simulink model "zynqRadioHWSWQPSKAD9361AD9364SL"  (R2016a)
settings: Solver=FixedStepDiscrete  SolverMode=SingleTasking  StartTime=0.0  StopTime=inf  RelTol=1e-3
PreLoadFcn:
  | % Ensure SDR libraries are added to path
  | tempradiodev_ = sdrdev('ZC706 and FMCOMMS2/3/4');
  | tempradiodev_.setupSession();
  | clear tempradiodev_; % clean up
  | 
  | sdrzQPSKTxFPGA_params = zynqRadioQPSKTxFPGAAD9361AD9364SL_init;
  | sdrzQPSKrxFPGA = zynqRadioQPSKRxFPGAAD9361AD9364SL_init;
  | 
  | % Need preamble & data from CST's QPSK Tx HDL example
  | qpsktxhdl=commqpsktxhdl_init();
  | 
  | % ARM Tx message
  | txtstr = '*Zynq HW/SW Codesign*';
InitFcn:
  | sdrzQPSKTxFPGA_params = zynqRadioQPSKTxFPGAAD9361AD9364SL_init;
  | sdrzQPSKrxFPGA = zynqRadioQPSKRxFPGAAD9361AD9364SL_init;
  | 
  | % Need preamble & data from CST's QPSK Tx HDL example
  | qpsktxhdl=commqpsktxhdl_init();
  | 
  | if (numel(txtstr) > 24)
  |   error('txtstr message must be less than 24 characters');
  | end;
undefined symbols (not defined in the file or in its folder): msglen
libraries: hdlsllib x9, dspsigops x7, commsequence2 x2, commdigbbndpm3 x2, dspmlti4 x2, commrandsrc2 x1, commutil2 x1, simulink x1, dspmathops x1
(part 1 of 2)
CloseFcn:
  | clear qpsktxhdl sdrzQPSKrxFPGA sdrzQPSKTxFPGA_params txtstr;
settings Model: DataTypeOverride=Off  Creator=The MathWorks, Inc.  LastModifiedBy=The MathWorks, Inc.
settings DataIOCC: SaveFormat=Array  SaveOutput=off  SaveTime=off
settings OptimizationCC: BlockReduction=off  ConditionallyExecuteInputs=off  DefaultParameterBehavior=Inlined
settings DebuggingCC: AlgebraicLoopMsg=error  SolverPrmCheckMsg=warning  SingleTaskRateTransMsg=error  ParameterPrecisionLossMsg=none  StrictBusMsg=ErrorOnBusTreatedAsVector
settings HardwareCC: ProdBitPerPointer=32  ProdLargestAtomicFloat=None  ProdIntDivRoundTo=Undefined  ProdEndianess=Unspecified  ProdWordSize=32  ProdHWDeviceType=ASIC/FPGA->ASIC/FPGA  ProdEqTarget=off
settings ModelReferenceCC: PropagateSignalLabelsOutOfModel=off

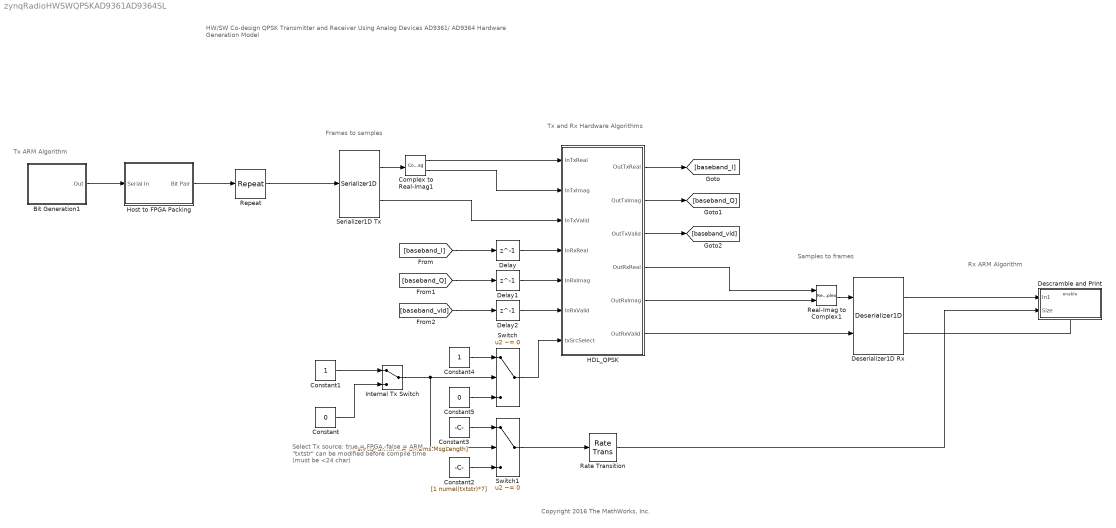
== system zynqRadioHWSWQPSKAD9361AD9364SL ==
  note: Select Tx source:
      | true = FPGA, false = ARM
      |
      | "txtstr" can be modified before
      | compile time (must be <24 char)
  note: Tx and Rx Hardware Algorithms
  note: HW/SW Co-design QPSK Transmitter and Receiver Using Analog Devices AD9361/ AD9364
      | Hardware Generation Model
  note: Rx ARM Algorithm
  note: Samples to frames
  note: Frames to samples
  note: Tx ARM Algorithm
  note: Copyright 2016 The MathWorks, Inc.
  Bit Generation1 : Subsystem
      mask Display: disp('Bits Generation')
  Complex to Real-Imag1 : ComplexToRealImag
  Constant : Constant  Value=0  OutDataTypeStr=boolean  SampleTime=-1
  Constant1 : Constant  OutDataTypeStr=boolean  SampleTime=-1
  Constant2 : Constant  Value=[1 numel(txtstr)*7]  SampleTime=-1
  Constant3 : Constant  Value=[1 sdrzQPSKTxFPGA_params.MsgLength]  SampleTime=-1
  Constant4 : Constant  OutDataTypeStr=boolean  SampleTime=-1
  Constant5 : Constant  Value=0  OutDataTypeStr=boolean  SampleTime=-1
  Delay : Delay  DelayLength=1
  Delay1 : Delay  DelayLength=1
  Delay2 : Delay  DelayLength=1
  Descramble and Print : Subsystem  TreatAsAtomicUnit=on
  Deserializer1D Rx : hdlsllib/HDL Operations/Deserializer1D  Ratio=sdrzQPSKrxFPGA.FrameSize  IdleCycles=0  InitialCondition=0  startIn=off  validIn=on  validOut=on  inputDataDimensions=-1  inputSampleTime=-1  inputSignalType=auto
  HDL_QPSK : Subsystem  TreatAsAtomicUnit=on
  Host to FPGA Packing : Subsystem
  Internal Tx Switch : ManualSwitch
  Rate Transition : RateTransition
  Real-Imag to Complex1 : RealImagToComplex
  Repeat : dspsigops/Repeat  N=4  InputProcessing=Columns as channels (frame based)  RateOptions=Allow multirate processing  ic=0  mode=Unused parameter value
  Serializer1D Tx : hdlsllib/HDL Operations/Serializer1D  Ratio=200  IdleCycles=0  validIn=off  startOut=off  validOut=on  inputDataDimensions=-1  inputSampleTime=-1  inputSignalType=auto
  Switch : Switch  Criteria=u2 ~= 0
  Switch1 : Switch  Criteria=u2 ~= 0
  wires:
  Deserializer1D Rx/1 -> Descramble and Print/1(In1)
  Real-Imag to Complex1/1 -> Deserializer1D Rx/1
  Deserializer1D Rx/2 -> Descramble and Print/Enable
  HDL_QPSK/4(OutRxReal) -> Real-Imag to Complex1/1
  HDL_QPSK/5(OutRxImag) -> Real-Imag to Complex1/2
  HDL_QPSK/6(OutRxValid) -> Deserializer1D Rx/2
  HDL_QPSK/1(OutTxReal) -> [baseband_I]
  HDL_QPSK/2(OutTxImag) -> [baseband_Q]
  HDL_QPSK/3(OutTxValid) -> [baseband_vld]
  [baseband_I] -> Delay/1
  [baseband_Q] -> Delay1/1
  [baseband_vld] -> Delay2/1
  Delay/1 -> HDL_QPSK/4(InRxReal)
  Delay1/1 -> HDL_QPSK/5(InRxImag)
  Delay2/1 -> HDL_QPSK/6(InRxValid)
  Host to FPGA Packing/1(Bit Pair) -> Repeat/1
  Bit Generation1/1(Out) -> Host to FPGA Packing/1(Serial In)
  Repeat/1 -> Serializer1D Tx/1
  Serializer1D Tx/1 -> Complex to Real-Imag1/1
  Complex to Real-Imag1/1 -> HDL_QPSK/1(InTxReal)
  Complex to Real-Imag1/2 -> HDL_QPSK/2(InTxImag)
  Serializer1D Tx/2 -> HDL_QPSK/3(InTxValid)
  Constant/1 -> Internal Tx Switch/2
  Constant1/1 -> Internal Tx Switch/1
  Switch1/1 -> Rate Transition/1
  Switch/1 -> HDL_QPSK/7(txSrcSelect)
  Internal Tx Switch/1 -> Switch1/2, Switch/2
  Constant4/1 -> Switch/1
  Constant5/1 -> Switch/3
  Constant2/1 -> Switch1/3
  Constant3/1 -> Switch1/1
  Rate Transition/1 -> Descramble and Print/2(Size)

== system zynqRadioHWSWQPSKAD9361AD9364SL/Bit Generation1 ==
  note: Each data frame contains 26 bits header (For Sync Purpose) and 174 bits data bits which
      | contain the txtStr message.Scrambler is there to improve data transition density and
      |  frequency offset estimation.
  Barker Code SS : Subsystem
      mask Display: disp('Unipolar\nBarker Code')
  Frame Conversion : FrameConversion  InheritSamplingMode=off  OutFrame=Sample-based
  Matrix Concatenate : Concatenate  Mode=Multidimensional array
  Message Source : Subsystem
      mask Display: disp('Message\nSource')
  Repeat : dspsigops/Repeat  N=2  InputProcessing=Columns as channels (frame based)  RateOptions=Enforce single-rate processing  ic=0  mode=Unused parameter value
  Scrambler : commsequence2/Scrambler  M=2  poly=[1 1 1 0 1]  iniStaSource=Dialog Parameter  ini_sta=[0 0 0 0]  resetViaPort=off
  Out : Outport
  wires:
  Message Source/1(Out) -> Scrambler/1
  Scrambler/1 -> Matrix Concatenate/2
  Repeat/1 -> Matrix Concatenate/1
  Barker Code SS/1(Out) -> Repeat/1
  Matrix Concatenate/1 -> Frame Conversion/1
  Frame Conversion/1 -> Out/1

== system zynqRadioHWSWQPSKAD9361AD9364SL/Descramble and Print ==
  In1 : Inport
  Size : Inport  Port=2
  Enable : EnablePort  PropagateVarSize=During execution
  BitsToDecimal1 : MATLAB Function  TreatAsAtomicUnit=on
  DataFramer : MATLAB Function  TreatAsAtomicUnit=on
  Descrambling : Subsystem
      mask Display: disp('Descrambling')
  wires:
  DataFramer/1(dataOut) -> Descrambling/1(In)
  In1/1 -> DataFramer/1(dataIn)
  Descrambling/1(Out) -> BitsToDecimal1/1(u)
  Size/1 -> Descrambling/2(Size)

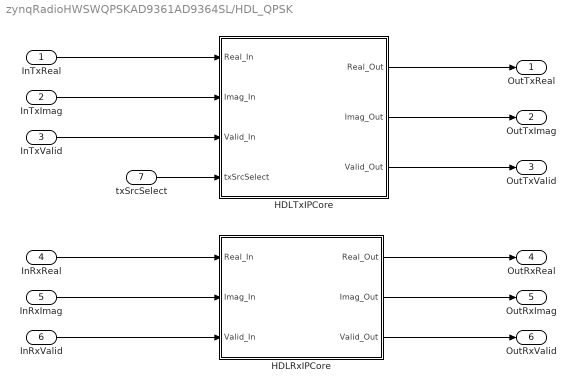
== system zynqRadioHWSWQPSKAD9361AD9364SL/HDL_QPSK ==
  InTxReal : Inport
  InTxImag : Inport  Port=2
  InTxValid : Inport  Port=3
  InRxReal : Inport  Port=4
  InRxImag : Inport  Port=5
  InRxValid : Inport  Port=6
  txSrcSelect : Inport  Port=7
  HDLRxIPCore : Subsystem  TreatAsAtomicUnit=on
  HDLTxIPCore : Subsystem  TreatAsAtomicUnit=on
  OutTxReal : Outport
  OutTxImag : Outport  Port=2
  OutTxValid : Outport  Port=3
  OutRxReal : Outport  Port=4
  OutRxImag : Outport  Port=5
  OutRxValid : Outport  Port=6
  wires:
  HDLTxIPCore/2(Imag_Out) -> OutTxImag/1
  InRxValid/1 -> HDLRxIPCore/3(Valid_In)
  HDLRxIPCore/3(Valid_Out) -> OutRxValid/1
  HDLRxIPCore/2(Imag_Out) -> OutRxImag/1
  HDLRxIPCore/1(Real_Out) -> OutRxReal/1
  HDLTxIPCore/3(Valid_Out) -> OutTxValid/1
  InRxImag/1 -> HDLRxIPCore/2(Imag_In)
  InRxReal/1 -> HDLRxIPCore/1(Real_In)
  HDLTxIPCore/1(Real_Out) -> OutTxReal/1
  InTxReal/1 -> HDLTxIPCore/1(Real_In)
  InTxImag/1 -> HDLTxIPCore/2(Imag_In)
  InTxValid/1 -> HDLTxIPCore/3(Valid_In)
  txSrcSelect/1 -> HDLTxIPCore/4(txSrcSelect)

== system zynqRadioHWSWQPSKAD9361AD9364SL/Host to FPGA Packing ==
  Serial In : Inport
  Data Type Conversion1 : DataTypeConversion  OutDataTypeStr=int16
  Downsample : DownSample  RateOptions=Allow multirate processing
  Downsample1 : DownSample  phase=1  RateOptions=Allow multirate processing
  Real-Imag to Complex : RealImagToComplex
  Bit Pair : Outport
  wires:
  Downsample/1 -> Real-Imag to Complex/1
  Serial In/1 -> Data Type Conversion1/1
  Data Type Conversion1/1 -> Downsample1/1, Downsample/1
  Downsample1/1 -> Real-Imag to Complex/2
  Real-Imag to Complex/1 -> Bit Pair/1

== system zynqRadioHWSWQPSKAD9361AD9364SL/Bit Generation1/Barker Code SS ==
  Constant Barker Code : Constant  Value=|  VectorParams1D=off  OutDataTypeStr=double
      | [+1 +1 +1 +1 +1 -1 -1 +1 +1 -1 +1 -1 +1
      | ].' > 0  % Bipolar to Unipolar Conversion
  Out : Outport
  wires:
  Constant Barker Code/1 -> Out/1

== system zynqRadioHWSWQPSKAD9361AD9364SL/Bit Generation1/Message Source ==
  Bernoulli Binary Generator : commrandsrc2/Bernoulli Binary Generator  P=0.5  seed=61  Ts=sdrzQPSKTxFPGA_params.FrameTime / (sdrzQPSKTxFPGA_params.DataLength - numel(txtstr)*7)  frameBased=on  sampPerFrame=sdrzQPSKTxFPGA_params.DataLength - numel(txtstr)*7  orient=off  outDataType=double
  Integer to Bit Converter : commutil2/Integer to Bit Converter  nbits=7  signedInputValues=Unsigned  bitOrder=MSB first  outDtype=Inherit via internal rule
  Matrix Concatenate : Concatenate  Mode=Multidimensional array
  Scroll text : Constant  Value=double(txtstr)
  Out : Outport
  wires:
  Matrix Concatenate/1 -> Out/1
  Bernoulli Binary Generator/1 -> Matrix Concatenate/2
  Integer to Bit Converter/1 -> Matrix Concatenate/1
  Scroll text/1 -> Integer to Bit Converter/1

== system zynqRadioHWSWQPSKAD9361AD9364SL/Descramble and Print/Descrambling ==
  In : Inport
  Size : Inport  Port=2
  Descrambler : commsequence2/Descrambler  M=2  poly=[1 1 1 0 1]  iniStaSource=Dialog Parameter  ini_sta=[0 0 0 0]  resetViaPort=off
  Selector : Selector  IndexOptions=Index vector (dialog)  Indices=[sdrzQPSKrxFPGA.BarkerLength*log2(sdrzQPSKrxFPGA.M)+1:sdrzQPSKrxFPGA.FrameSize*log2(sdrzQPSKrxFPGA.M)]  OutputSizes=1
  Selector1 : Selector  IndexOptions=Starting and ending indices (port)  Indices=[1:msglen]  OutputSizes=1
  Out : Outport
  wires:
  Selector/1 -> Descrambler/1
  In/1 -> Selector/1
  Selector1/1 -> Out/1
  Descrambler/1 -> Selector1/1
  Size/1 -> Selector1/2

== system zynqRadioHWSWQPSKAD9361AD9364SL/HDL_QPSK/HDLRxIPCore ==
  Real_In : Inport
  Imag_In : Inport  Port=2
  Valid_In : Inport  Port=3
  Complex to Real-Imag1 : ComplexToRealImag
  Enabled Delay : Delay  DelayLength=1  ShowEnablePort=on
      settings: InputPortMap=u0,e6
  HDLRx : Subsystem
  Real-Imag to Complex : RealImagToComplex
  Repeat : dspsigops/Repeat  N=sdrzQPSKrxFPGA.Upsampling/sdrzQPSKrxFPGA.Downsampling  InputProcessing=Inherited (this choice will be removed - see release notes)  RateOptions=Allow multirate processing  ic=0  mode=Unused parameter value
  Upsample : dspsigops/Upsample  N=sdrzQPSKrxFPGA.Upsampling/sdrzQPSKrxFPGA.Downsampling  phase=0  InputProcessing=Inherited (this choice will be removed - see release notes)  RateOptions=Allow multirate processing  ic=0  mode=Unused parameter value
  Real_Out : Outport
  Imag_Out : Outport  Port=2
  Valid_Out : Outport  Port=3
  wires:
  HDLRx/2(dValidOut) -> Upsample/1
  Upsample/1 -> Valid_Out/1
  Repeat/1 -> Complex to Real-Imag1/1
  Complex to Real-Imag1/1 -> Real_Out/1
  Valid_In/1 -> Enabled Delay/2
  Complex to Real-Imag1/2 -> Imag_Out/1
  HDLRx/1(dataOutCh1) -> Repeat/1
  Real-Imag to Complex/1 -> Enabled Delay/1
  Enabled Delay/1 -> HDLRx/1(dataInCh1)
  Real_In/1 -> Real-Imag to Complex/1
  Imag_In/1 -> Real-Imag to Complex/2

== system zynqRadioHWSWQPSKAD9361AD9364SL/HDL_QPSK/HDLTxIPCore ==
  Real_In : Inport
  Imag_In : Inport  Port=2
  Valid_In : Inport  Port=3
  txSrcSelect : Inport  Port=4
  Complex to Real-Imag1 : ComplexToRealImag
  Delay : Delay  DelayLength=1
  Enabled Delay : Delay  DelayLength=1  ShowEnablePort=on
      settings: InputPortMap=u0,e6
  HDLTx : Subsystem
  Real-Imag to Complex : RealImagToComplex
  Real_Out : Outport
  Imag_Out : Outport  Port=2
  Valid_Out : Outport  Port=3
  wires:
  Complex to Real-Imag1/1 -> Real_Out/1
  Complex to Real-Imag1/2 -> Imag_Out/1
  HDLTx/1(dataoutCh1) -> Complex to Real-Imag1/1
  HDLTx/2(validoutCh1) -> Valid_Out/1
  Real-Imag to Complex/1 -> Enabled Delay/1
  Valid_In/1 -> HDLTx/2(validInCh1), Enabled Delay/2
  Real_In/1 -> Real-Imag to Complex/1
  Imag_In/1 -> Real-Imag to Complex/2
  Enabled Delay/1 -> HDLTx/1(dataInCh1)
  txSrcSelect/1 -> Delay/1
  Delay/1 -> HDLTx/3(txSrcSelect)

== system zynqRadioHWSWQPSKAD9361AD9364SL/HDL_QPSK/HDLRxIPCore/HDLRx ==
  dataInCh1 : Inport
  Automatic Gain Control : Subsystem  mask{AGCLoopGain=0.1, AGCUpperLimit=400, AGCRef=1/sqrt(sdrzQPSKrxFPGA.Upsampling)}
      mask prompts: AGCLoopGain "Loop Gain"; AGCUpperLimit "Maximum Gain"; AGCRef "Desired Amplitude"
  Coarse Frequency Compensation : Subsystem
  Data Decoding : Subsystem  TreatAsAtomicUnit=on  mask{Threshold=16}
      mask help:
      | Package synchronization is achieved by correlating (matched filtering) the Barker codes with the streams given by the Timing Recovery subsystem.
      | We deem successful package synchronization if the modulus of the matched filter output exceeds the threshold value defined below.
  FPGA to Host : Subsystem
  Fine Frequency Compensation : Subsystem
  Logical Operator1 : Logic  AllPortsSameDT=off  OutDataTypeStr=boolean
  Raised Cosine Receive Filter : dspmlti4/FIR Decimation  FilterSource=Dialog parameters  h=sdrzQPSKrxFPGA.ReceiverFilterCoefficients  D=sdrzQPSKrxFPGA.Upsampling/sdrzQPSKrxFPGA.Downsampling  filtStruct=Direct form  FilterObject=Hm_firdecim  framing=Allow multirate processing  inputOffset=0  outputBufInitCond=0  roundingMode=Floor  overflowMode=off  firstCoeffDataTypeStr=Inherit: Same word length as input  firstCoeffMin=[]  firstCoeffMax=[]  firstCoeffLastDataTypeStr=Inherit: Same word length as input  outputMode=Binary point scaling  outputWordLength=16  outputFracLength=14  outputDataTypeStr=fixdt(1,16,14)  outputMin=[]  outputMax=[]  outputLastDataTypeStr=fixdt(1,16,14)
  Timing Recovery : Subsystem
  dataOutCh1 : Outport
  dValidOut : Outport  Port=2
  wires:
  Logical Operator1/1 -> dValidOut/1
  Raised Cosine Receive Filter/1 -> Coarse Frequency Compensation/1(In)
  Automatic Gain Control/1(Out) -> Raised Cosine Receive Filter/1
  FPGA to Host/1(Out) -> dataOutCh1/1
  Data Decoding/2(Bit1) -> FPGA to Host/1(bit1)
  Data Decoding/3(Bit2) -> FPGA to Host/2(bit2)
  Data Decoding/1(dValid) -> Logical Operator1/2
  Timing Recovery/1(dValid) -> Data Decoding/Enable, Logical Operator1/1
  Coarse Frequency Compensation/1(Out) -> Fine Frequency Compensation/1(In)
  Fine Frequency Compensation/1(Out) -> Timing Recovery/1(In)
  dataInCh1/1 -> Automatic Gain Control/1(In)
  Timing Recovery/2(DataOut) -> Data Decoding/1(In)

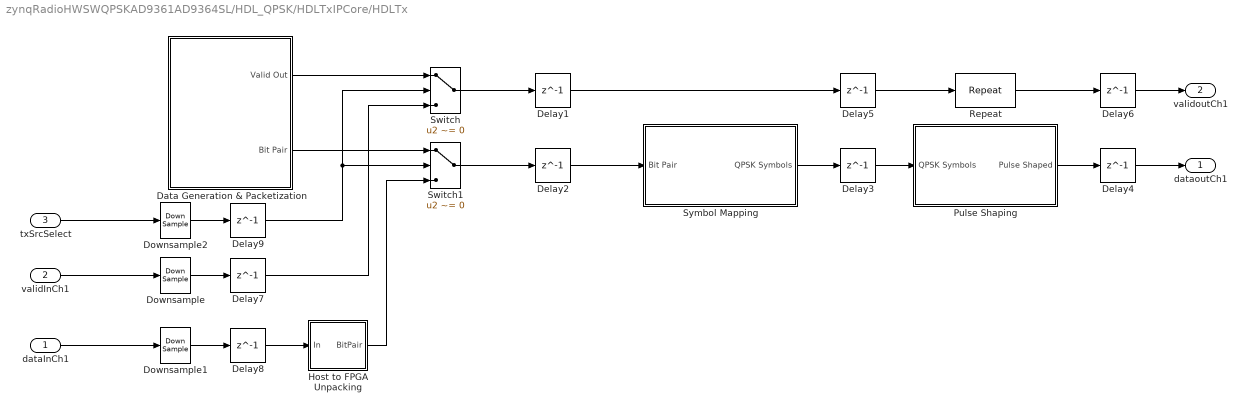
== system zynqRadioHWSWQPSKAD9361AD9364SL/HDL_QPSK/HDLTxIPCore/HDLTx ==
  dataInCh1 : Inport
  validInCh1 : Inport  Port=2
  txSrcSelect : Inport  Port=3
  Data Generation & Packetization : Subsystem
  Delay{1..9} (9 alike) : Delay  DelayLength=1  InitialCondition=0
  Downsample : DownSample  N=sdrzQPSKTxFPGA_params.Upsampling  RateOptions=Allow multirate processing
  Downsample1 : DownSample  N=sdrzQPSKTxFPGA_params.Upsampling  RateOptions=Allow multirate processing
  Downsample2 : DownSample  N=sdrzQPSKTxFPGA_params.Upsampling  RateOptions=Allow multirate processing
  Host to FPGA Unpacking : Subsystem
  Pulse Shaping : Subsystem
  Repeat : dspsigops/Repeat  N=sdrzQPSKTxFPGA_params.Upsampling  InputProcessing=Inherited (this choice will be removed - see release notes)  RateOptions=Allow multirate processing  ic=0  mode=Unused parameter value
  Switch : Switch  Criteria=u2 ~= 0
  Switch1 : Switch  Criteria=u2 ~= 0
  Symbol Mapping : Subsystem
  dataoutCh1 : Outport
  validoutCh1 : Outport  Port=2
  wires:
  Delay3/1 -> Pulse Shaping/1(QPSK Symbols)
  Pulse Shaping/1(Pulse Shaped) -> Delay4/1
  Delay4/1 -> dataoutCh1/1
  Delay2/1 -> Symbol Mapping/1(Bit Pair)
  Symbol Mapping/1(QPSK Symbols) -> Delay3/1
  Delay1/1 -> Delay5/1
  Delay5/1 -> Repeat/1
  Repeat/1 -> Delay6/1
  Delay6/1 -> validoutCh1/1
  Data Generation & Packetization/1(Valid Out) -> Switch/1
  Data Generation & Packetization/2(Bit Pair) -> Switch1/1
  Switch/1 -> Delay1/1
  Switch1/1 -> Delay2/1
  Downsample/1 -> Delay7/1
  Downsample1/1 -> Delay8/1
  validInCh1/1 -> Downsample/1
  dataInCh1/1 -> Downsample1/1
  Delay8/1 -> Host to FPGA Unpacking/1(In)
  Host to FPGA Unpacking/1(BitPair) -> Switch1/3
  Delay7/1 -> Switch/3
  Downsample2/1 -> Delay9/1
  txSrcSelect/1 -> Downsample2/1
  Delay9/1 -> Switch/2, Switch1/2

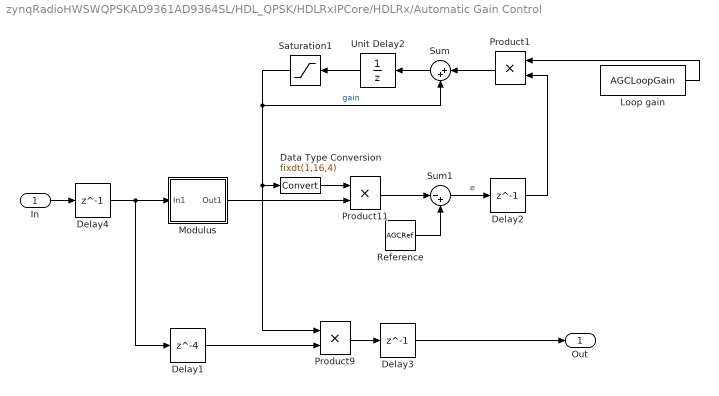
== system zynqRadioHWSWQPSKAD9361AD9364SL/HDL_QPSK/HDLRxIPCore/HDLRx/Automatic Gain Control ==
  In : Inport
  Data Type Conversion : DataTypeConversion  OutDataTypeStr=fixdt(1,16,4)  SaturateOnIntegerOverflow=on
  Delay1 : Delay  DelayLength=4  InitialCondition=0
  Delay2 : Delay  DelayLength=1  InitialCondition=0
  Delay3 : Delay  DelayLength=1  InitialCondition=0
  Delay4 : Delay  DelayLength=1  InitialCondition=0
  Loop gain : Constant  Value=AGCLoopGain  OutDataTypeStr=fixdt(1,16,10)  SampleTime=sdrzQPSKrxFPGA.Ts
  Modulus : Subsystem
  Product1 : Product  OutDataTypeStr=fixdt(1,16,10)  RndMeth=Zero
  Product11 : Product  OutDataTypeStr=fixdt(1,16,10)  RndMeth=Zero
  Product9 : Product  OutDataTypeStr=fixdt(1,16,14)  SaturateOnIntegerOverflow=on  RndMeth=Zero
  Reference : Constant  Value=AGCRef  OutDataTypeStr=fixdt(1,16,10)  SampleTime=sdrzQPSKrxFPGA.Ts
  Saturation1 : Saturate  UpperLimit=AGCUpperLimit  LowerLimit=1e-5
  Sum : Sum  Inputs=|++  OutDataTypeStr=fixdt(1,23,10)  SaturateOnIntegerOverflow=on
  Sum1 : Sum  Inputs=|-+  OutDataTypeStr=Inherit: Same as first input
  Unit Delay2 : UnitDelay  SampleTime=-1
  Out : Outport  PortDimensions=1
  wires:
  Loop gain/1 -> Product1/1
  Saturation1/1 -> Product9/1, Data Type Conversion/1, Sum/2  "gain"
  Product1/1 -> Sum/1
  Modulus/1(Out1) -> Product11/2
  Delay4/1 -> Modulus/1(In1), Delay1/1
  Unit Delay2/1 -> Saturation1/1
  Delay2/1 -> Product1/2
  Delay3/1 -> Out/1
  Delay1/1 -> Product9/2
  Product9/1 -> Delay3/1
  Sum1/1 -> Delay2/1  "e"
  Sum/1 -> Unit Delay2/1
  Reference/1 -> Sum1/2
  Data Type Conversion/1 -> Product11/1
  Product11/1 -> Sum1/1
  In/1 -> Delay4/1

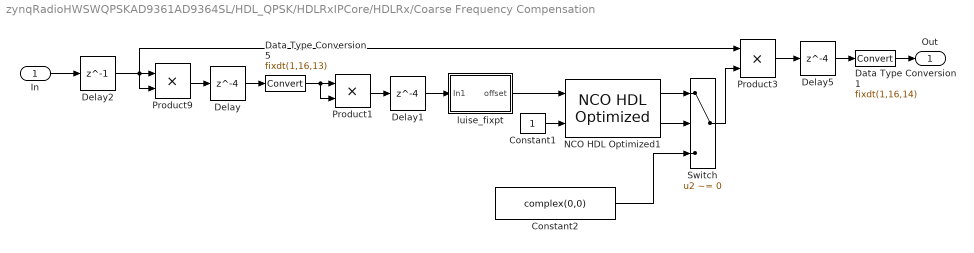
== system zynqRadioHWSWQPSKAD9361AD9364SL/HDL_QPSK/HDLRxIPCore/HDLRx/Coarse Frequency Compensation ==
  In : Inport  PortDimensions=1
  Constant1 : Constant  OutDataTypeStr=boolean  SampleTime=sdrzQPSKrxFPGA.Ts*sdrzQPSKrxFPGA.Upsampling/sdrzQPSKrxFPGA.Downsampling
  Constant2 : Constant  Value=complex(0,0)  OutDataTypeStr=fixdt(1,10,8)  SampleTime=sdrzQPSKrxFPGA.Ts*sdrzQPSKrxFPGA.Upsampling/sdrzQPSKrxFPGA.Downsampling
  Data Type Conversion1 : DataTypeConversion  OutDataTypeStr=fixdt(1,16,14)
  Data Type Conversion5 : DataTypeConversion  OutDataTypeStr=fixdt(1,16,13)  SaturateOnIntegerOverflow=on
  Delay : Delay  DelayLength=4  InitialCondition=0
  Delay1 : Delay  DelayLength=4  InitialCondition=0
  Delay2 : Delay  DelayLength=1  InitialCondition=0
  Delay5 : Delay  DelayLength=4  InitialCondition=0
  NCO HDL Optimized1 : dspsigops/NCO HDL Optimized  PhaseIncrementSource=Input port  PhaseIncrement=100  PhaseOffsetSource=Property  PhaseOffset=0  DitherSource=None  NumDitherBits=1  PhaseQuantization=on  NumQuantizerAccumulatorBits=16  LUTCompress=on  ResetAction=off  ValidInputPort=on  Waveform=Complex exponential  PhasePort=off  AccumulatorWL=17  OutputDataType=Binary point scaling  OutputWL=10  OutputFL=8  SimulateUsing=Code generation
  Product1 : Product  SaturateOnIntegerOverflow=on  RndMeth=Zero
  Product3 : Product  SaturateOnIntegerOverflow=on  RndMeth=Zero
  Product9 : Product  SaturateOnIntegerOverflow=on  RndMeth=Zero
  Switch : Switch  Criteria=u2 ~= 0
  luise_fixpt : Subsystem
  Out : Outport
  wires:
  luise_fixpt/1(offset) -> NCO HDL Optimized1/1
  Delay2/1 -> Product9/1, Product9/2, Product3/1
  Switch/1 -> Product3/2
  Constant2/1 -> Switch/3
  NCO HDL Optimized1/1 -> Switch/1
  NCO HDL Optimized1/2 -> Switch/2
  Constant1/1 -> NCO HDL Optimized1/2
  Delay5/1 -> Data Type Conversion1/1
  Product3/1 -> Delay5/1
  In/1 -> Delay2/1
  Product1/1 -> Delay1/1
  Data Type Conversion5/1 -> Product1/2, Product1/1
  Delay/1 -> Data Type Conversion5/1
  Product9/1 -> Delay/1
  Delay1/1 -> luise_fixpt/1(In1)
  Data Type Conversion1/1 -> Out/1

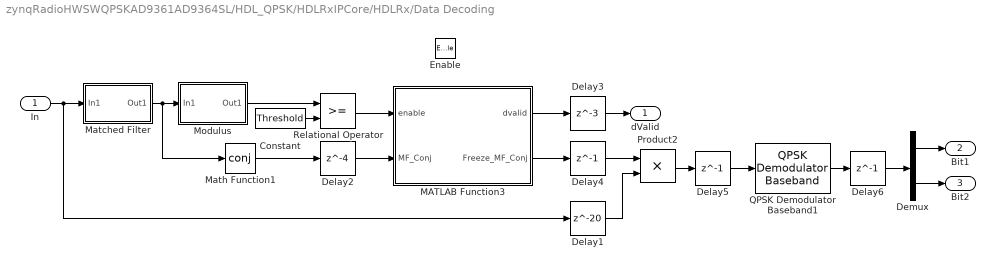
== system zynqRadioHWSWQPSKAD9361AD9364SL/HDL_QPSK/HDLRxIPCore/HDLRx/Data Decoding ==
  In : Inport
  Enable : EnablePort
  Constant : Constant  Value=Threshold  OutDataTypeStr=Inherit: Inherit via back propagation  SampleTime=sdrzQPSKrxFPGA.Ts*sdrzQPSKrxFPGA.Upsampling/sdrzQPSKrxFPGA.Downsampling
  Delay1 : Delay  DelayLength=20  InitialCondition=0
  Delay2 : Delay  DelayLength=4  InitialCondition=0
  Delay3 : Delay  DelayLength=3  InitialCondition=0
  Delay4 : Delay  DelayLength=1  InitialCondition=0
  Delay5 : Delay  DelayLength=1  InitialCondition=0
  Delay6 : Delay  DelayLength=1  InitialCondition=0
  Demux : Demux  Outputs=2
  MATLAB Function3 : MATLAB Function  TreatAsAtomicUnit=on
  Matched Filter : Subsystem
  Math Function1 : Math  Operator=conj  OutputSignalType=complex  SaturateOnIntegerOverflow=on
  Modulus : Subsystem
  Product2 : Product  SaturateOnIntegerOverflow=on  RndMeth=Zero
  QPSK Demodulator Baseband1 : commdigbbndpm3/QPSK Demodulator Baseband  OutType=Bit  DecType=Hard decision  VarSource=Dialog  Variance=1  Dec=Gray  Ph=pi/4  outDtype1=boolean  outDtype2=Inherit via internal rule  derotateFactorWordLen=16  derotateFactorDataTypeStr=Inherit: Same word length as input  derotateFactorLastDataTypeStr=Inherit: Same word length as input
  Relational Operator : RelationalOperator  OutDataTypeStr=boolean  InputSameDT=on
  dValid : Outport  InitialOutput=0
  Bit1 : Outport  Port=2  InitialOutput=0
  Bit2 : Outport  Port=3  InitialOutput=0
  wires:
  Constant/1 -> Relational Operator/2
  Modulus/1(Out1) -> Relational Operator/1
  QPSK Demodulator Baseband1/1 -> Delay6/1
  MATLAB Function3/1(dvalid) -> Delay3/1
  MATLAB Function3/2(Freeze_MF_Conj) -> Delay4/1
  Math Function1/1 -> Delay2/1
  Relational Operator/1 -> MATLAB Function3/1(enable)
  Product2/1 -> Delay5/1
  In/1 -> Matched Filter/1(In1), Delay1/1
  Matched Filter/1(Out1) -> Modulus/1(In1), Math Function1/1
  Delay2/1 -> MATLAB Function3/2(MF_Conj)
  Delay4/1 -> Product2/1
  Delay1/1 -> Product2/2
  Delay5/1 -> QPSK Demodulator Baseband1/1
  Delay6/1 -> Demux/1
  Delay3/1 -> dValid/1
  Demux/1 -> Bit1/1
  Demux/2 -> Bit2/1

== system zynqRadioHWSWQPSKAD9361AD9364SL/HDL_QPSK/HDLRxIPCore/HDLRx/FPGA to Host ==
  bit1 : Inport
  bit2 : Inport  Port=2
  Data Type Conversion1 : DataTypeConversion  OutDataTypeStr=int16
  Data Type Conversion2 : DataTypeConversion  OutDataTypeStr=int16
  Real-Imag to Complex : RealImagToComplex
  Out : Outport
  wires:
  bit1/1 -> Data Type Conversion1/1
  Data Type Conversion2/1 -> Real-Imag to Complex/2
  bit2/1 -> Data Type Conversion2/1
  Real-Imag to Complex/1 -> Out/1
  Data Type Conversion1/1 -> Real-Imag to Complex/1

== system zynqRadioHWSWQPSKAD9361AD9364SL/HDL_QPSK/HDLRxIPCore/HDLRx/Fine Frequency Compensation ==
  In : Inport  PortDimensions=1
  Delay2 : Delay  DelayLength=1  InitialCondition=0
  Delay5 : Delay  DelayLength=9  InitialCondition=0
  Loop Filter : Subsystem  mask{BnTs=0.06, zeta=2.5, N=sdrzQPSKrxFPGA.Upsampling/sdrzQPSKrxFPGA.Downsampling, Kp=sdrzQPSKrxFPGA.FineFreqPEDGain, K0=sdrzQPSKrxFPGA.FineFreqCompensateGain}
      mask prompts: BnTs "Normalized Loop Bandwidth"; zeta "Damping Factor"; N "Number of Samples/Symbol"; Kp "Phase Detector Gain (Kp)"; K0 "DDS Gain (K0)"
      mask init:
      | % See C.57 to C.61 in Michael Rice's "Digital Communications 
      | % - A Discrete-Time Approach" for details
      | theta = BnTs/(zeta+0.25/zeta)/N;
      | d = 1 + 2*zeta*theta + theta*theta;
      | K1 = 4*zeta*theta/d;
      | K2 = 4*theta*theta/d;
      | K1 = K1/(Kp*K0);
      | K2 = K2/(Kp*K0);
      mask Display: disp('Loop Filter')
  MATLAB Function1 : MATLAB Function  TreatAsAtomicUnit=on
  NCO : Subsystem
  Product9 : Product  OutDataTypeStr=fixdt(1,16,14)  SaturateOnIntegerOverflow=on  RndMeth=Zero
  Out : Outport
  wires:
  Loop Filter/1(v) -> NCO/1(In1)
  Delay2/1 -> MATLAB Function1/1(In), Out/1
  NCO/1(Out1) -> Product9/2
  MATLAB Function1/1(e) -> Loop Filter/1(e)
  Product9/1 -> Delay2/1
  Delay5/1 -> Product9/1
  In/1 -> Delay5/1

== system zynqRadioHWSWQPSKAD9361AD9364SL/HDL_QPSK/HDLRxIPCore/HDLRx/Timing Recovery ==
  In : Inport
  Delay5 : Delay  DelayLength=6
  Integer Delay3 : Delay  DelayLength=1  InputProcessing=Inherited
  Integer Delay4 : Delay  DelayLength=1  InputProcessing=Inherited
  Interpolation Control : MATLAB Function
  Interpolation Filter : Subsystem
  Loop Filter : Subsystem  mask{BnTs=0.01, zeta=1, Kp=sdrzQPSKrxFPGA.TimingRecTEDGain, K0=sdrzQPSKrxFPGA.TimingRecCompensateGain, N=sdrzQPSKrxFPGA.Upsampling/sdrzQPSKrxFPGA.Downsampling}
      mask prompts: BnTs "Loop Bandwidth"; zeta "Loop Damping Factor"; Kp "Phase Detector Gain (Kp)"; K0 "DDS gain (K0)"; N "Number of Samples/symbol (N)"
      mask init:
      | % See C.57 to C.61 in Michael Rice's "Digital Communications 
      | % - A Discrete-Time Approach" for details
      | theta = BnTs/(zeta+0.25/zeta)/N;
      | d = 1 + 2*zeta*theta + theta*theta;
      | K1 = 4*zeta*theta/d;
      | K2 = 4*theta*theta/d;
      | K1 = K1/(Kp*K0);
      | K2 = K2/(Kp*K0);
      mask Display: disp('Loop Filter');
  Timing Error Detector : MATLAB Function  TreatAsAtomicUnit=on
  dValid : Outport
  DataOut : Outport  Port=2
  wires:
  Loop Filter/1(v) -> Interpolation Control/1(Delta)
  Timing Error Detector/1(e) -> Loop Filter/1(e)
  Integer Delay3/1 -> dValid/1, Timing Error Detector/2(strobe)
  Delay5/1 -> Interpolation Filter/1(In)
  Interpolation Control/1(Underflow) -> Integer Delay3/1
  Interpolation Control/2(mu) -> Integer Delay4/1
  Integer Delay4/1 -> Interpolation Filter/2(mu)
  In/1 -> Delay5/1
  Interpolation Filter/1(Out) -> DataOut/1, Timing Error Detector/1(In)

== system zynqRadioHWSWQPSKAD9361AD9364SL/HDL_QPSK/HDLTxIPCore/HDLTx/Data Generation & Packetization ==
  Bit Pairing : Subsystem
  Data Source : Subsystem
  Downsample : DownSample  RateOptions=Allow multirate processing
  PacketizerFSM : MATLAB Function  TreatAsAtomicUnit=on  SystemSampleTime=1/sdrzQPSKrxFPGA.RadioFrontEndSampleRate*2
  Pipeline : Delay  InitialCondition=0
  Pipeline1 : Delay  DelayLength=1  InitialCondition=0
  Pipeline2 : Delay  DelayLength=1  InitialCondition=0
  Pipeline3 : Delay  DelayLength=1  InitialCondition=0
  Valid : Constant  OutDataTypeStr=boolean  SampleTime=1/sdrzQPSKrxFPGA.RadioFrontEndSampleRate*2
  Valid Out : Outport
  Bit Pair : Outport  Port=2
  wires:
  Bit Pairing/1(Bit Pair) -> Bit Pair/1
  Pipeline2/1 -> Bit Pairing/1(Serial In)
  Data Source/1(packets) -> Pipeline2/1
  Valid/1 -> Pipeline/1
  Pipeline1/1 -> Downsample/1
  Pipeline/1 -> Pipeline1/1
  Downsample/1 -> Pipeline3/1
  Pipeline3/1 -> Valid Out/1
  PacketizerFSM/1(reset_preamble) -> Data Source/1(reset preamble)
  PacketizerFSM/2(load_preamble) -> Data Source/2(load preamble)
  PacketizerFSM/3(load_data) -> Data Source/3(load data)

== system zynqRadioHWSWQPSKAD9361AD9364SL/HDL_QPSK/HDLTxIPCore/HDLTx/Host to FPGA Unpacking ==
  In : Inport
  Bit Concat : hdlsllib/HDL Operations/Bit Concat  numInputs=2
  Bit Slice1 : hdlsllib/HDL Operations/Bit Slice  lidx=0  ridx=0
  Bit Slice2 : hdlsllib/HDL Operations/Bit Slice  lidx=0  ridx=0
  Complex to Real-Imag : ComplexToRealImag
  BitPair : Outport
  wires:
  Complex to Real-Imag/1 -> Bit Slice2/1
  Complex to Real-Imag/2 -> Bit Slice1/1
  Bit Slice2/1 -> Bit Concat/1
  Bit Slice1/1 -> Bit Concat/2
  Bit Concat/1 -> BitPair/1
  In/1 -> Complex to Real-Imag/1

== system zynqRadioHWSWQPSKAD9361AD9364SL/HDL_QPSK/HDLTxIPCore/HDLTx/Pulse Shaping ==
  QPSK Symbols : Inport
  RRC Interpolation Filter : dspmlti4/FIR Interpolation  FilterSource=Dialog parameters  h=sdrzQPSKTxFPGA_params.TransmitterFilterCoefficients  L=sdrzQPSKTxFPGA_params.Upsampling  FilterObject=Htxrc  framing=Allow multirate processing  outputBufInitCond=0  roundingMode=Floor  overflowMode=off  firstCoeffMode=Specify word length  firstCoeffWordLength=16  firstCoeffFracLength=15  firstCoeffDataTypeStr=fixdt(1,16)  firstCoeffMin=[]  firstCoeffMax=[]  firstCoeffLastDataTypeStr=fixdt(1,16)  prodOutputMode=Binary point scaling  prodOutputWordLength=31  prodOutputFracLength=29  prodOutputDataTypeStr=fixdt(1,31,29)  prodOutputLastDataTypeStr=fixdt(1,31,29)  accumMode=Binary point scaling  accumWordLength=33  accumFracLength=29  accumDataTypeStr=fixdt(1,33,29)  accumLastDataTypeStr=fixdt(1,33,29)  outputMode=Binary point scaling  outputWordLength=16  outputFracLength=14  outputDataTypeStr=fixdt(1,16,14)  outputMin=[]  outputMax=[]  outputLastDataTypeStr=fixdt(1,16,14)
  Pulse Shaped : Outport
  wires:
  QPSK Symbols/1 -> RRC Interpolation Filter/1
  RRC Interpolation Filter/1 -> Pulse Shaped/1

== system zynqRadioHWSWQPSKAD9361AD9364SL/HDL_QPSK/HDLTxIPCore/HDLTx/Symbol Mapping ==
  Bit Pair : Inport
  QPSK Modulator Baseband : commdigbbndpm3/QPSK Modulator Baseband  InType=Integer  Enc=Gray  Ph=pi/4  outDtype=Fixed-point  outWordLen=16  outUDDataType=sfix(16)  outFracLenMode=User-defined  outFracLen=15  outDataTypeStr=fixdt(1,16,15)  outLastDataTypeStr=fixdt(1,16,15)
  QPSK Symbols : Outport
  wires:
  QPSK Modulator Baseband/1 -> QPSK Symbols/1
  Bit Pair/1 -> QPSK Modulator Baseband/1

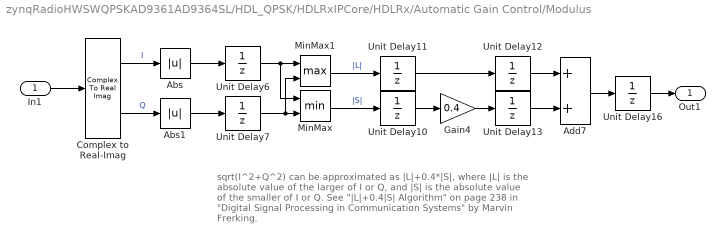
== system zynqRadioHWSWQPSKAD9361AD9364SL/HDL_QPSK/HDLRxIPCore/HDLRx/Automatic Gain Control/Modulus ==
  note: sqrt(I^2+Q^2) can be approximated as |L|+0.4*|S|,
      | where |L| is the absolute value of the larger of I or Q,
      | and |S| is the absolute value of the smaller of I or Q.
      |
      | See "|L|+0.4|S| Algorithm" on page 238 in "Digital Signal
      | Processing in Communication Systems" by Marvin Frerking.
  In1 : Inport
  Abs : Abs
  Abs1 : Abs
  Add7 : Sum
  Complex to Real-Imag : ComplexToRealImag
  Gain4 : Gain  Gain=0.4  OutDataTypeStr=fixdt(1,16,15)
  MinMax : MinMax  Inputs=2
  MinMax1 : MinMax  Function=max  Inputs=2
  Unit Delay{6..7,10..13,16} (7 alike) : UnitDelay  SampleTime=-1
  Out1 : Outport
  wires:
  In1/1 -> Complex to Real-Imag/1
  Unit Delay7/1 -> MinMax/2, MinMax1/2
  Unit Delay6/1 -> MinMax1/1, MinMax/1
  MinMax/1 -> Unit Delay10/1  "|S|"
  Gain4/1 -> Unit Delay13/1
  Unit Delay13/1 -> Add7/2
  MinMax1/1 -> Unit Delay11/1  "|L|"
  Complex to Real-Imag/2 -> Abs1/1  "Q"
  Complex to Real-Imag/1 -> Abs/1  "I"
  Abs/1 -> Unit Delay6/1
  Add7/1 -> Unit Delay16/1
  Abs1/1 -> Unit Delay7/1
  Unit Delay12/1 -> Add7/1
  Unit Delay10/1 -> Gain4/1
  Unit Delay16/1 -> Out1/1
  Unit Delay11/1 -> Unit Delay12/1

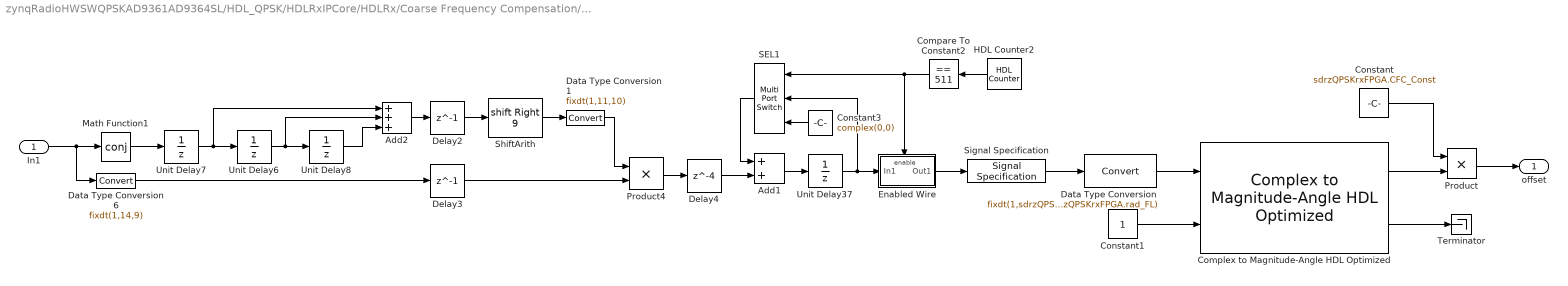
== system zynqRadioHWSWQPSKAD9361AD9364SL/HDL_QPSK/HDLRxIPCore/HDLRx/Coarse Frequency Compensation/luise_fixpt ==
  In1 : Inport
  Add1 : Sum  OutDataTypeStr=fixdt(1,33,20)
  Add2 : Sum  Inputs=+++  OutDataTypeStr=fixdt(1,33,20)
  Compare To Constant2 : simulink/Logic and Bit Operations/Compare To Constant  relop===  const=511  OutDataTypeStr=boolean
  Complex to Magnitude-Angle HDL Optimized : dspmathops/Complex to Magnitude-Angle HDL Optimized  NumIterationsSource=Property  NumIterations=5  OutputFormat=Angle  AngleFormat=Normalized  ScaleOutput=on  SimulateUsing=Code generation
  Constant : Constant  Value=sdrzQPSKrxFPGA.CFC_Const  OutDataTypeStr=int16  SampleTime=sdrzQPSKrxFPGA.Ts*sdrzQPSKrxFPGA.Upsampling/sdrzQPSKrxFPGA.Downsampling
  Constant1 : Constant  OutDataTypeStr=boolean  SampleTime=sdrzQPSKrxFPGA.Ts*sdrzQPSKrxFPGA.Upsampling/sdrzQPSKrxFPGA.Downsampling
  Constant3 : Constant  Value=complex(0,0)  OutDataTypeStr=fixdt(1,16,14)  SampleTime=sdrzQPSKrxFPGA.Ts*sdrzQPSKrxFPGA.Upsampling/sdrzQPSKrxFPGA.Downsampling
  Data Type Conversion : DataTypeConversion  OutDataTypeStr=fixdt(1,sdrzQPSKrxFPGA.rad_WL,sdrzQPSKrxFPGA.rad_FL)
  Data Type Conversion1 : DataTypeConversion  OutDataTypeStr=fixdt(1,11,10)
  Data Type Conversion6 : DataTypeConversion  OutDataTypeStr=fixdt(1,14,9)  SaturateOnIntegerOverflow=on
  Delay2 : Delay  DelayLength=1  InitialCondition=0
  Delay3 : Delay  DelayLength=1  InitialCondition=0
  Delay4 : Delay  DelayLength=4  InitialCondition=0
  Enabled Wire : Subsystem  TreatAsAtomicUnit=on
  HDL Counter2 : hdlsllib/HDL Operations/HDL Counter  CountType=Count limited  CountInit=0  CountStep=1  CountMax=511  CountFromType=Initial value  CountFrom=0  CountResetPort=off  CountLoadPort=off  CountEnbPort=off  CountDirPort=off  CountDataType=Unsigned  CountWordLen=9  CountFracLen=0  CountSampTime=-1
  Math Function1 : Math  Operator=conj  OutputSignalType=complex  SaturateOnIntegerOverflow=on
  Product : Product  OutDataTypeStr=int16
  Product4 : Product  SaturateOnIntegerOverflow=on  RndMeth=Zero
  SEL1 : MultiPortSwitch  DataPortOrder=Zero-based contiguous  Inputs=2  DiagnosticForDefault=None  OutDataTypeStr=fixdt(1,33,20)
  ShiftArith : ArithShift  BitShiftNumber=9  BitShiftDirection=Right
  Signal Specification : SignalSpecification  Dimensions=1
  Terminator : Terminator
  Unit Delay37 : UnitDelay  InitialCondition=0+0j  SampleTime=-1
  Unit Delay6 : UnitDelay  SampleTime=-1
  Unit Delay7 : UnitDelay  SampleTime=-1
  Unit Delay8 : UnitDelay  SampleTime=-1
  offset : Outport  PortDimensions=1
  wires:
  Data Type Conversion/1 -> Complex to Magnitude-Angle HDL Optimized/1
  Complex to Magnitude-Angle HDL Optimized/2 -> Terminator/1
  Signal Specification/1 -> Data Type Conversion/1
  Constant1/1 -> Complex to Magnitude-Angle HDL Optimized/2
  Complex to Magnitude-Angle HDL Optimized/1 -> Product/2
  Constant/1 -> Product/1
  Product/1 -> offset/1
  Enabled Wire/1(Out1) -> Signal Specification/1
  Add1/1 -> Unit Delay37/1
  Math Function1/1 -> Unit Delay7/1
  Product4/1 -> Delay4/1
  In1/1 -> Math Function1/1, Data Type Conversion6/1
  Data Type Conversion1/1 -> Product4/1
  Delay4/1 -> Add1/2
  Unit Delay37/1 -> SEL1/2, Enabled Wire/1(In1)
  SEL1/1 -> Add1/1
  Add2/1 -> Delay2/1
  Data Type Conversion6/1 -> Delay3/1
  Constant3/1 -> SEL1/3
  Unit Delay6/1 -> Unit Delay8/1, Add2/2
  Unit Delay7/1 -> Add2/1, Unit Delay6/1
  Compare To Constant2/1 -> SEL1/1, Enabled Wire/Enable
  HDL Counter2/1 -> Compare To Constant2/1
  Unit Delay8/1 -> Add2/3
  ShiftArith/1 -> Data Type Conversion1/1
  Delay3/1 -> Product4/2
  Delay2/1 -> ShiftArith/1

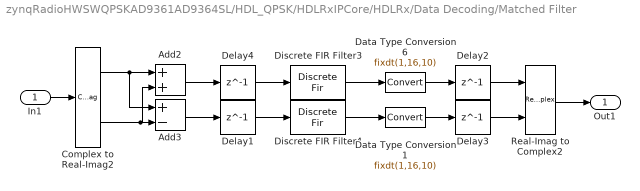
== system zynqRadioHWSWQPSKAD9361AD9364SL/HDL_QPSK/HDLRxIPCore/HDLRx/Data Decoding/Matched Filter ==
  In1 : Inport
  Add2 : Sum
  Add3 : Sum  Inputs=+-
  Complex to Real-Imag2 : ComplexToRealImag
  Data Type Conversion1 : DataTypeConversion  OutDataTypeStr=fixdt(1,16,10)
  Data Type Conversion6 : DataTypeConversion  OutDataTypeStr=fixdt(1,16,10)
  Delay{1..4} (4 alike) : Delay  DelayLength=1  InitialCondition=0
  Discrete FIR Filter3 : DiscreteFir  FilterStructure=Direct form transposed  Coefficients=[-1 1 -1 1 -1 -1 1 1 -1 -1 -1 -1 -1]
  Discrete FIR Filter4 : DiscreteFir  FilterStructure=Direct form transposed  Coefficients=-1*[-1 1 -1 1 -1 -1 1 1 -1 -1 -1 -1 -1]
  Real-Imag to Complex2 : RealImagToComplex
  Out1 : Outport
  wires:
  In1/1 -> Complex to Real-Imag2/1
  Real-Imag to Complex2/1 -> Out1/1
  Complex to Real-Imag2/2 -> Add3/2, Add2/2
  Complex to Real-Imag2/1 -> Add2/1, Add3/1
  Data Type Conversion1/1 -> Delay3/1
  Add2/1 -> Delay4/1
  Data Type Conversion6/1 -> Delay2/1
  Add3/1 -> Delay1/1
  Discrete FIR Filter3/1 -> Data Type Conversion6/1
  Delay4/1 -> Discrete FIR Filter3/1
  Discrete FIR Filter4/1 -> Data Type Conversion1/1
  Delay2/1 -> Real-Imag to Complex2/1
  Delay3/1 -> Real-Imag to Complex2/2
  Delay1/1 -> Discrete FIR Filter4/1

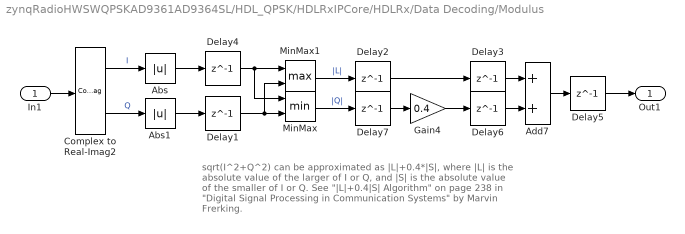
== system zynqRadioHWSWQPSKAD9361AD9364SL/HDL_QPSK/HDLRxIPCore/HDLRx/Data Decoding/Modulus ==
  note: sqrt(I^2+Q^2) can be approximated as |L|+0.4*|S|,
      | where |L| is the absolute value of the larger of I or Q,
      | and |S| is the absolute value of the smaller of I or Q.
      |
      | See "|L|+0.4|S| Algorithm" on page 238 in "Digital Signal
      | Processing in Communication Systems" by Marvin Frerking.
  In1 : Inport
  Abs : Abs
  Abs1 : Abs
  Add7 : Sum
  Complex to Real-Imag2 : ComplexToRealImag
  Delay{1..7} (7 alike) : Delay  DelayLength=1  InitialCondition=0
  Gain4 : Gain  Gain=0.4  OutDataTypeStr=fixdt(1,16,15)
  MinMax : MinMax  Inputs=2
  MinMax1 : MinMax  Function=max  Inputs=2
  Out1 : Outport
  wires:
  In1/1 -> Complex to Real-Imag2/1
  Abs1/1 -> Delay1/1
  Abs/1 -> Delay4/1
  Gain4/1 -> Delay6/1
  MinMax1/1 -> Delay2/1  "|L|"
  MinMax/1 -> Delay7/1  "|Q|"
  Add7/1 -> Delay5/1
  Delay7/1 -> Gain4/1
  Delay2/1 -> Delay3/1
  Delay1/1 -> MinMax1/2, MinMax/2
  Delay4/1 -> MinMax1/1, MinMax/1
  Delay6/1 -> Add7/2
  Delay5/1 -> Out1/1
  Delay3/1 -> Add7/1
  Complex to Real-Imag2/2 -> Abs1/1  "Q"
  Complex to Real-Imag2/1 -> Abs/1  "I"

== system zynqRadioHWSWQPSKAD9361AD9364SL/HDL_QPSK/HDLRxIPCore/HDLRx/Fine Frequency Compensation/Loop Filter ==
  note: Proportional-plus-Integrator Loop Filter,
      | Infinite DC Response to guarantee convergence
  e : Inport
  Data Type Conversion3 : DataTypeConversion  OutDataTypeStr=fixdt(1,32,29)
  Delay1 : Delay  DelayLength=1  InitialCondition=0
  Delay2 : Delay  DelayLength=1  InitialCondition=0
  Digital Filter : Subsystem
  K1 : Gain  Gain=K1
  K2 : Gain  Gain=K2
  Sum2 : Sum  OutDataTypeStr=fixdt(1,22,19)  SaturateOnIntegerOverflow=on  InputSameDT=on
  v : Outport
  wires:
  Delay1/1 -> v/1
  Digital Filter/1(Out1) -> Sum2/2
  Sum2/1 -> Delay1/1
  K2/1 -> Digital Filter/1(In1)
  Data Type Conversion3/1 -> Sum2/1
  Delay2/1 -> K2/1, K1/1
  e/1 -> Delay2/1
  K1/1 -> Data Type Conversion3/1

== system zynqRadioHWSWQPSKAD9361AD9364SL/HDL_QPSK/HDLRxIPCore/HDLRx/Fine Frequency Compensation/NCO ==
  In1 : Inport
  Constant : Constant  Value=sdrzQPSKrxFPGA.FFC_Const  OutDataTypeStr=int16  SampleTime=sdrzQPSKrxFPGA.Ts*sdrzQPSKrxFPGA.Upsampling/sdrzQPSKrxFPGA.Downsampling
  Constant1 : Constant  OutDataTypeStr=boolean  SampleTime=sdrzQPSKrxFPGA.Ts*sdrzQPSKrxFPGA.Upsampling/sdrzQPSKrxFPGA.Downsampling
  Constant2 : Constant  Value=complex(0,0)  OutDataTypeStr=fixdt(1,10,8)  SampleTime=sdrzQPSKrxFPGA.Ts*sdrzQPSKrxFPGA.Upsampling/sdrzQPSKrxFPGA.Downsampling
  Delay3 : Delay  DelayLength=1  InitialCondition=0
  NCO HDL Optimized : dspsigops/NCO HDL Optimized  PhaseIncrementSource=Input port  PhaseIncrement=100  PhaseOffsetSource=Property  PhaseOffset=0  DitherSource=None  NumDitherBits=1  PhaseQuantization=on  NumQuantizerAccumulatorBits=16  LUTCompress=on  ResetAction=off  ValidInputPort=on  Waveform=Complex exponential  PhasePort=off  AccumulatorWL=17  OutputDataType=Binary point scaling  OutputWL=10  OutputFL=8  SimulateUsing=Code generation
  Product : Product  OutDataTypeStr=int16
  Signal Specification : SignalSpecification  Dimensions=1
  Switch : Switch  Criteria=u2 ~= 0
  Out1 : Outport
  wires:
  Delay3/1 -> Out1/1
  Constant2/1 -> Switch/3
  NCO HDL Optimized/2 -> Switch/2
  Constant1/1 -> NCO HDL Optimized/2
  NCO HDL Optimized/1 -> Switch/1
  Signal Specification/1 -> NCO HDL Optimized/1
  Switch/1 -> Delay3/1
  Product/1 -> Signal Specification/1
  Constant/1 -> Product/2
  In1/1 -> Product/1

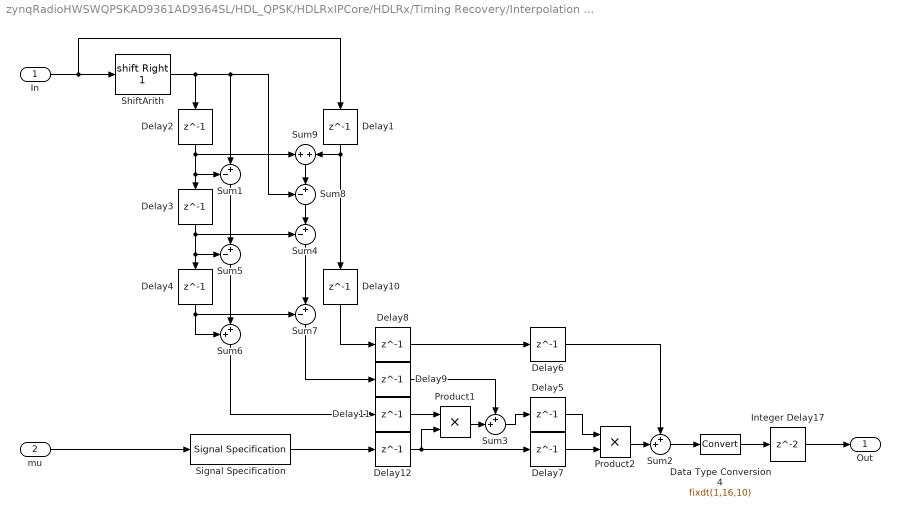
== system zynqRadioHWSWQPSKAD9361AD9364SL/HDL_QPSK/HDLRxIPCore/HDLRx/Timing Recovery/Interpolation Filter ==
  In : Inport
  mu : Inport  Port=2
  Data Type Conversion4 : DataTypeConversion  OutDataTypeStr=fixdt(1,16,10)
  Delay{1..12} (12 alike) : Delay  DelayLength=1  InitialCondition=0
  Integer Delay17 : Delay  InputProcessing=Inherited
  Product1 : Product  OutDataTypeStr=fixdt(1,16,10)  RndMeth=Zero
  Product2 : Product  RndMeth=Zero
  ShiftArith : ArithShift  BitShiftNumber=1  BitShiftDirection=Right
  Signal Specification : SignalSpecification  Dimensions=1
  Sum{1,4..5,8} (4 alike) : Sum  Inputs=-+|
  Sum2 : Sum  Inputs=++|
  Sum3 : Sum  Inputs=++|  OutDataTypeStr=fixdt(1,16,10)
  Sum6 : Sum  Inputs=++|  OutDataTypeStr=fixdt(1,16,11)  SaturateOnIntegerOverflow=on
  Sum7 : Sum  Inputs=-+|  OutDataTypeStr=fixdt(1,16,10)
  Sum9 : Sum  Inputs=+|+
  Out : Outport
  wires:
  Signal Specification/1 -> Delay12/1
  Sum9/1 -> Sum8/2
  Data Type Conversion4/1 -> Integer Delay17/1
  In/1 -> ShiftArith/1, Delay1/1
  Integer Delay17/1 -> Out/1
  mu/1 -> Signal Specification/1
  Sum6/1 -> Delay11/1
  Sum7/1 -> Delay9/1
  Delay10/1 -> Delay8/1
  Delay6/1 -> Sum2/1
  Delay7/1 -> Product2/2
  Delay12/1 -> Product1/2, Delay7/1
  Delay8/1 -> Delay6/1
  Delay9/1 -> Sum3/1
  Delay11/1 -> Product1/1
  Sum2/1 -> Data Type Conversion4/1
  Product1/1 -> Sum3/2
  Product2/1 -> Sum2/2
  Sum3/1 -> Delay5/1
  Delay5/1 -> Product2/1
  Sum4/1 -> Sum7/2
  Sum5/1 -> Sum6/2
  Delay4/1 -> Sum7/1, Sum6/1
  Sum1/1 -> Sum5/2
  Delay3/1 -> Sum4/1, Sum5/1, Delay4/1
  Sum8/1 -> Sum4/2
  Delay2/1 -> Sum1/1, Delay3/1, Sum9/1
  Delay1/1 -> Delay10/1, Sum9/2
  ShiftArith/1 -> Sum8/1, Sum1/2, Delay2/1

== system zynqRadioHWSWQPSKAD9361AD9364SL/HDL_QPSK/HDLRxIPCore/HDLRx/Timing Recovery/Loop Filter ==
  note: Proportional-Plus-Integrator Loop Filter,
      | Infinite DC Response to guarantee convergence
  e : Inport
  Data Type Conversion17 : DataTypeConversion  OutDataTypeStr=fixdt(1,11,10)
  Delay1 : Delay  DelayLength=1  InitialCondition=0
  Delay2 : Delay  DelayLength=1  InitialCondition=0
  Delay4 : Delay  DelayLength=1  InitialCondition=0
  Digital Filter : Subsystem
  K1 : Gain  Gain=K1  OutDataTypeStr=fixdt(1,40,33)
  K2 : Gain  Gain=K2
  Sum2 : Sum  SaturateOnIntegerOverflow=on  InputSameDT=on
  v : Outport
  wires:
  K1/1 -> Delay1/1
  Digital Filter/1(Out1) -> Delay4/1
  K2/1 -> Digital Filter/1(In1)
  Data Type Conversion17/1 -> v/1
  Delay2/1 -> K2/1, K1/1
  Delay4/1 -> Sum2/2
  Delay1/1 -> Sum2/1
  Sum2/1 -> Data Type Conversion17/1
  e/1 -> Delay2/1

== system zynqRadioHWSWQPSKAD9361AD9364SL/HDL_QPSK/HDLTxIPCore/HDLTx/Data Generation & Packetization/Bit Pairing ==
  Serial In : Inport
  Bit Concat : hdlsllib/HDL Operations/Bit Concat  numInputs=2
  Delay1 : Delay  DelayLength=1
  Delay2 : Delay  DelayLength=1
  Downsample : DownSample  phase=1  RateOptions=Allow multirate processing
  Downsample1 : DownSample  RateOptions=Allow multirate processing
  Bit Pair : Outport
  wires:
  Downsample1/1 -> Delay1/1
  Serial In/1 -> Downsample1/1, Downsample/1
  Bit Concat/1 -> Bit Pair/1
  Downsample/1 -> Delay2/1
  Delay1/1 -> Bit Concat/2
  Delay2/1 -> Bit Concat/1

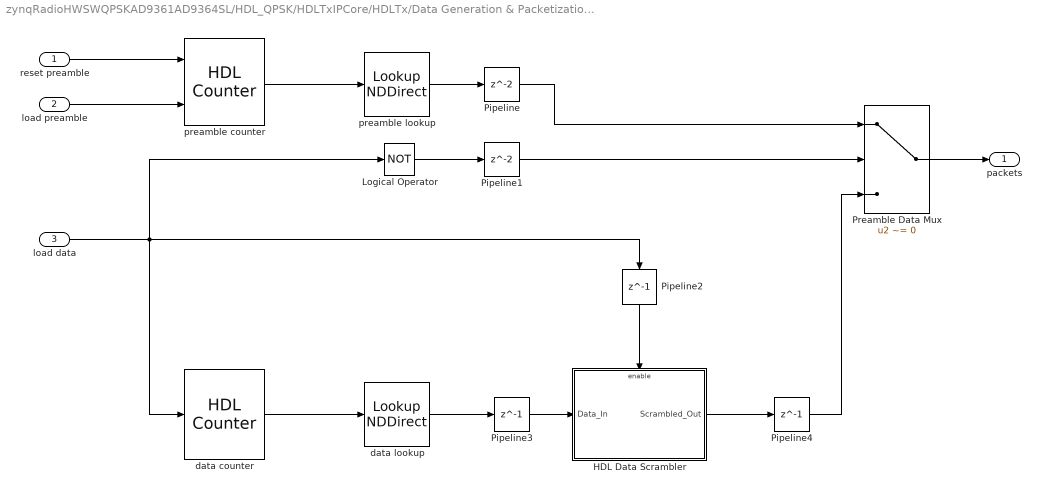
== system zynqRadioHWSWQPSKAD9361AD9364SL/HDL_QPSK/HDLTxIPCore/HDLTx/Data Generation & Packetization/Data Source ==
  reset preamble : Inport
  load preamble : Inport  Port=2
  load data : Inport  Port=3
  HDL Data Scrambler : Subsystem  TreatAsAtomicUnit=on
  Logical Operator : Logic  Operator=NOT  AllPortsSameDT=off  OutDataTypeStr=boolean
  Pipeline : Delay  InitialCondition=0
  Pipeline1 : Delay  InitialCondition=0
  Pipeline2 : Delay  DelayLength=1  InitialCondition=0
  Pipeline3 : Delay  DelayLength=1  InitialCondition=0
  Pipeline4 : Delay  DelayLength=1  InitialCondition=0
  Preamble Data Mux : Switch  Criteria=u2 ~= 0
  data counter : hdlsllib/HDL Operations/HDL Counter  CountType=Count limited  CountInit=0  CountStep=1  CountMax=17399  CountFromType=Initial value  CountFrom=0  CountResetPort=off  CountLoadPort=off  CountEnbPort=on  CountDirPort=off  CountDataType=Unsigned  CountWordLen=16  CountFracLen=0  CountSampTime=1
  data lookup : LookupNDDirect  NumberOfTableDimensions=1  Table=[qpsktxhdl.data]  DiagnosticForOutOfRangeInput=Error  TableDataTypeStr=boolean
  preamble counter : hdlsllib/HDL Operations/HDL Counter  CountType=Free running  CountInit=0  CountStep=1  CountMax=256  CountFromType=Initial value  CountFrom=0  CountResetPort=on  CountLoadPort=off  CountEnbPort=on  CountDirPort=off  CountDataType=Unsigned  CountWordLen=8  CountFracLen=0  CountSampTime=1
  preamble lookup : LookupNDDirect  NumberOfTableDimensions=1  Table=[qpsktxhdl.preamble]  DiagnosticForOutOfRangeInput=Error  TableDataTypeStr=boolean
  packets : Outport
  wires:
  load data/1 -> data counter/1, Pipeline2/1, Logical Operator/1
  Logical Operator/1 -> Pipeline1/1
  Pipeline2/1 -> HDL Data Scrambler/Enable
  Preamble Data Mux/1 -> packets/1
  Pipeline1/1 -> Preamble Data Mux/2
  Pipeline/1 -> Preamble Data Mux/1
  Pipeline4/1 -> Preamble Data Mux/3
  Pipeline3/1 -> HDL Data Scrambler/1(Data_In)
  preamble lookup/1 -> Pipeline/1
  HDL Data Scrambler/1(Scrambled_Out) -> Pipeline4/1
  data lookup/1 -> Pipeline3/1
  data counter/1 -> data lookup/1
  reset preamble/1 -> preamble counter/1
  load preamble/1 -> preamble counter/2
  preamble counter/1 -> preamble lookup/1

== system zynqRadioHWSWQPSKAD9361AD9364SL/HDL_QPSK/HDLRxIPCore/HDLRx/Coarse Frequency Compensation/luise_fixpt/Enabled Wire ==
  In1 : Inport
  Enable : EnablePort
  Data Type Conversion : DataTypeConversion  OutDataTypeStr=fixdt(1,sdrzQPSKrxFPGA.rad_WL,sdrzQPSKrxFPGA.rad_FL)
  Out1 : Outport  InitialOutput=0
  wires:
  In1/1 -> Data Type Conversion/1
  Data Type Conversion/1 -> Out1/1

== system zynqRadioHWSWQPSKAD9361AD9364SL/HDL_QPSK/HDLRxIPCore/HDLRx/Fine Frequency Compensation/Loop Filter/Digital Filter ==
  In1 : Inport
  Add1 : Sum  OutDataTypeStr=fixdt(1,32,29)
  Unit Delay1 : UnitDelay  SampleTime=-1
  Out1 : Outport
  wires:
  Unit Delay1/1 -> Add1/1
  Add1/1 -> Out1/1, Unit Delay1/1
  In1/1 -> Add1/2

== system zynqRadioHWSWQPSKAD9361AD9364SL/HDL_QPSK/HDLRxIPCore/HDLRx/Timing Recovery/Loop Filter/Digital Filter ==
  In1 : Inport
  Add2 : Sum  OutDataTypeStr=fixdt(1,40,33)
  Unit Delay1 : UnitDelay  SampleTime=-1
  Out1 : Outport
  wires:
  Unit Delay1/1 -> Add2/1
  Add2/1 -> Out1/1, Unit Delay1/1
  In1/1 -> Add2/2

== system zynqRadioHWSWQPSKAD9361AD9364SL/HDL_QPSK/HDLTxIPCore/HDLTx/Data Generation & Packetization/Data Source/HDL Data Scrambler ==
  note: HDL optimized scrambler, implementing the scrambler
      | polynomial [1 1 1 0 1], with initial states [0 0 0 0]
  Data_In : Inport
  Enable : EnablePort
  BIT_XOR : Logic  Operator=XOR  IconShape=distinctive  AllPortsSameDT=off  OutDataTypeStr=boolean
  BIT_XOR1 : Logic  Operator=XOR  IconShape=distinctive  AllPortsSameDT=off  OutDataTypeStr=boolean
  BIT_XOR2 : Logic  Operator=XOR  IconShape=distinctive  AllPortsSameDT=off  OutDataTypeStr=boolean
  p{1..4} (4 alike) : Delay  DelayLength=1
  Scrambled_Out : Outport  InitialOutput=0
  wires:
  BIT_XOR2/1 -> p1/1, Scrambled_Out/1
  p4/1 -> BIT_XOR/2
  p1/1 -> p2/1, BIT_XOR1/1
  BIT_XOR/1 -> BIT_XOR1/2
  p3/1 -> p4/1
  p2/1 -> p3/1, BIT_XOR/1
  BIT_XOR1/1 -> BIT_XOR2/2
  Data_In/1 -> BIT_XOR2/1

== matlab function zynqRadioHWSWQPSKAD9361AD9364SL/Descramble and Print/BitsToDecimal1 ==
  data: u input
function BitsToASCII(u)
%#codegen
% Convert bits to ASCII message.
% Convert binary-valued column vector to 7-bit decimal values.
w = [64 32 16 8 4 2 1]; % binary digit weighting
Nbits = numel(u);
Ny = Nbits/7;
y = zeros(1,Ny);
for i = 0:Ny-1
    y(i+1) = w*u(7*i+(1:7));
end

% replace the non-printable characters with "^" char(94) 
% to indicate an error 
y(y > 126)= 94; 
y(y < 32) = 94;
% Display ASCII message to command window
fprintf('%s\n',char(y));

== matlab function zynqRadioHWSWQPSKAD9361AD9364SL/HDL_QPSK/HDLRxIPCore/HDLRx/Data Decoding/MATLAB Function3 ==
  data: dvalid output; Freeze_MF_Conj output; enable input; MF_Conj input
function [dvalid,Freeze_MF_Conj] = fcn(enable,MF_Conj)
%#codegen

persistent state;
persistent counter;
persistent MF_Out_Reg;

if isempty(state);
    state      = false;
    counter    = uint8(0);
    MF_Out_Reg = complex(fi(0,1,16,10),fi(0,1,16,10));
end

Freeze_MF_Conj = MF_Out_Reg;

if state==false
    dvalid=false;
else %state==true
    dvalid=true;
    counter = counter-1;         
end


% state transition
if state==false && enable==true
    state=true;
    counter=uint8(100);
    MF_Out_Reg=MF_Conj;
elseif state==true && counter==0
    if enable==true % packages come back-to-back
        state      = true;
        counter    = uint8(100);
        MF_Out_Reg = MF_Conj;
    else
        state = false;    
    end
end

== matlab function zynqRadioHWSWQPSKAD9361AD9364SL/HDL_QPSK/HDLRxIPCore/HDLRx/Fine Frequency Compensation/MATLAB Function1 ==
  data: In input; e output
function e  = PED(In)
% Input:
%   In - Input samples, oversampled by two
% Output:
%   e - Phase error
% PED implements 
% e = sign(real(In)).*imag(In) - sign(imag(In)).*real(In);

%#codegen

OP2 = real(In);
OP1 = imag(In);

Real = OP2;
Imag = OP1;

if (bitget(Real,16)==true) % real component is negative
    OP1 = fi(-Imag,1,16,14);
end
if (bitget(Imag,16)==true) % imaginary component is negative
    OP2 = fi(-Real,1,16,14);
end

e= fi(OP1-OP2,1,16,14);
